simulink library "Library_SII"  (R2014b)
settings: Solver=ode45  StartTime=0.0  StopTime=10.0  RelTol=1e-3
libraries: fl_lib x77, Library_SII x44, nesl_utility x33, powerlib x15, mblibv1 x11, simulink x6, elec_lib x5, powerlib_extras x1
(part 3 of 4)

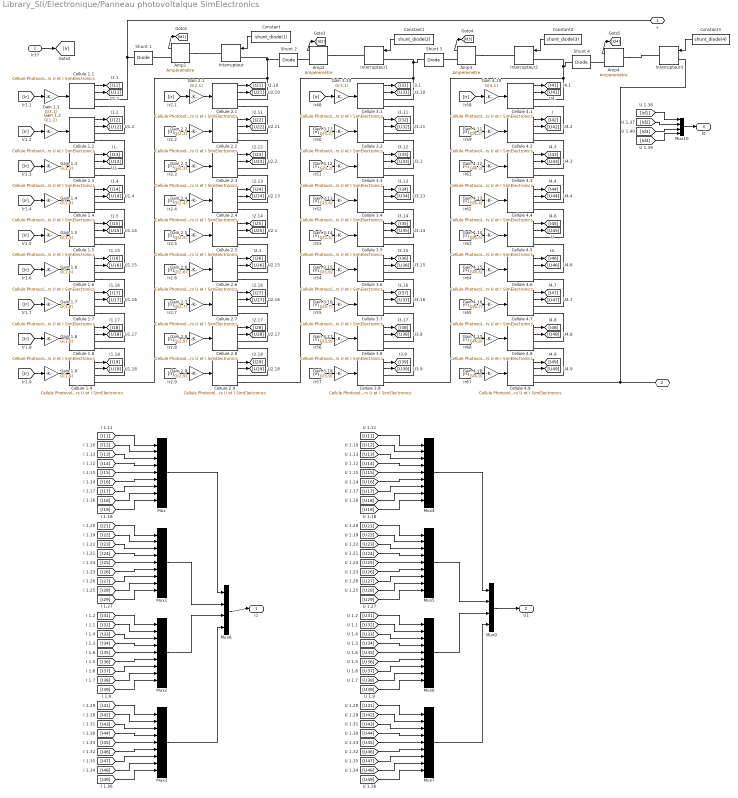
== system Library_SII/Electronique/Panneau photovoltaique SimElectronics ==
  Ir37 : Inport
  Amp{1..4} (4 alike) : Library_SII/Electronique/Ampèremètre
  Cellule 1.1 : Library_SII/Electronique/Cellule Photovoltaique avec capteurs U et I SimElectronics  typcell=polycristallin  Icc=Icc  Vco=Vco  Tcell=Tcell  shunt=0  mesure=off  IRef=1000  TRef=25  Qf=1.4
  Cellule 1.{2..8} (7 alike) : Library_SII/Electronique/Cellule Photovoltaique avec capteurs U et I SimElectronics  typcell=polycristallin  Icc=Icc  Vco=Vco  Tcell=Tcell  shunt=0  mesure=off  IRef=1000  TRef=25  Qf=1.5
  Cellule 1.9 : Library_SII/Electronique/Cellule Photovoltaique avec capteurs U et I SimElectronics  typcell=polycristallin  Icc=Icc  Vco=Vco  Tcell=Tcell  shunt=1  mesure=off  IRef=1000  TRef=25  Qf=1.5
  Cellule 2.{1..7} (7 alike) : Library_SII/Electronique/Cellule Photovoltaique avec capteurs U et I SimElectronics  typcell=polycristallin  Icc=Icc  Vco=Vco  Tcell=Tcell  shunt=0  mesure=off  IRef=1000  TRef=25  Qf=1.5
  Cellule 2.8 : Library_SII/Electronique/Cellule Photovoltaique avec capteurs U et I SimElectronics  typcell=polycristallin  Icc=Icc  Vco=Vco  Tcell=Tcell  shunt=0  mesure=off  IRef=1000  TRef=25  Qf=10
  Cellule 2.9 : Library_SII/Electronique/Cellule Photovoltaique avec capteurs U et I SimElectronics  typcell=polycristallin  Icc=Icc  Vco=Vco  Tcell=Tcell  shunt=1  mesure=off  IRef=1000  TRef=25  Qf=1.5
  Cellule 3.{1..8} (8 alike) : Library_SII/Electronique/Cellule Photovoltaique avec capteurs U et I SimElectronics  typcell=polycristallin  Icc=Icc  Vco=Vco  Tcell=Tcell  shunt=0  mesure=off  IRef=1000  TRef=25  Qf=1.5
  Cellule 3.9 : Library_SII/Electronique/Cellule Photovoltaique avec capteurs U et I SimElectronics  typcell=polycristallin  Icc=Icc  Vco=Vco  Tcell=Tcell  shunt=1  mesure=off  IRef=1000  TRef=25  Qf=1.5
  Cellule 4.{1..8} (8 alike) : Library_SII/Electronique/Cellule Photovoltaique avec capteurs U et I SimElectronics  typcell=polycristallin  Icc=Icc  Vco=Vco  Tcell=Tcell  shunt=0  mesure=off  IRef=1000  TRef=25  Qf=1.5
  Cellule 4.9 : Library_SII/Electronique/Cellule Photovoltaique avec capteurs U et I SimElectronics  typcell=polycristallin  Icc=Icc  Vco=Vco  Tcell=Tcell  shunt=1  mesure=off  IRef=1000  TRef=25  Qf=1.5
  Constant : Constant  Value=shunt_diode(1)
  Constant1 : Constant  Value=shunt_diode(2)
  Constant2 : Constant  Value=shunt_diode(3)
  Constant3 : Constant  Value=shunt_diode(4)
  Gain 1.1 : Gain  Gain=G(1,1)
  Gain 1.2 : Gain  Gain=G(1,2)
  Gain 1.3 : Gain  Gain=G(1,3)
  Gain 1.4 : Gain  Gain=G(1,4)
  Gain 1.5 : Gain  Gain=G(1,5)
  Gain 1.6 : Gain  Gain=G(1,6)
  Gain 1.7 : Gain  Gain=G(1,7)
  Gain 1.8 : Gain  Gain=G(1,8)
  Gain 1.9 : Gain  Gain=G(1,9)
  Gain 2.1 : Gain  Gain=G(2,1)
  Gain 2.2 : Gain  Gain=G(2,2)
  Gain 2.3 : Gain  Gain=G(2,3)
  Gain 2.4 : Gain  Gain=G(2,4)
  Gain 2.5 : Gain  Gain=G(2,5)
  Gain 2.6 : Gain  Gain=G(2,6)
  Gain 2.7 : Gain  Gain=G(2,7)
  Gain 2.8 : Gain  Gain=G(2,8)
  Gain 2.9 : Gain  Gain=G(2,9)
  Gain 3.10 : Gain  Gain=G(3,1)
  Gain 3.11 : Gain  Gain=G(3,2)
  Gain 3.12 : Gain  Gain=G(3,3)
  Gain 3.13 : Gain  Gain=G(3,4)
  Gain 3.14 : Gain  Gain=G(3,5)
  Gain 3.15 : Gain  Gain=G(3,6)
  Gain 3.16 : Gain  Gain=G(3,7)
  Gain 3.17 : Gain  Gain=G(3,8)
  Gain 3.18 : Gain  Gain=G(3,9)
  Gain 4.10 : Gain  Gain=G(4,1)
  Gain 4.11 : Gain  Gain=G(4,2)
  Gain 4.12 : Gain  Gain=G(4,3)
  Gain 4.13 : Gain  Gain=G(4,4)
  Gain 4.14 : Gain  Gain=G(4,5)
  Gain 4.15 : Gain  Gain=G(4,6)
  Gain 4.16 : Gain  Gain=G(4,7)
  Gain 4.17 : Gain  Gain=G(4,8)
  Gain 4.18 : Gain  Gain=G(4,9)
  Interrupteur{,1..3} (4 alike) : Library_SII/Electronique/Interrupteur
  Mux{,1..7} (8 alike) : Mux  Inputs=9
  Mux10 : Mux
  Mux8 : Mux
  Mux9 : Mux
  Shunt {1..4} (4 alike) : elec_lib/Semiconductor Devices/Diode  ModelType=1  Vf=0.6 V  Ron=0.3 Ohm  Goff=1e-8 S  Rz=0.3 Ohm  Vz=50 V  C_PWL=5 pF  prmExp=1  I12=[ 0.0137 0.545 ] A  V12=[ 0.6 0.7 ] V  I1=0.0137 A  V1=0.6 V  RS=0.01 Ohm  IS=1e-12 A  Tmeas=25 C  ec=1  BV=Inf V  C_param=1  CJ0=5 pF  VJ=1 V  Mgrad=0.5  Vvec=[ 0.1 10 100 ] V  Cvec=[ 3.5 1 0.4 ] pF  FC=0.5  Q_param=1  Irrm=-7.15 A  iF=4 A  didt=-750 A/us  trr=115 ns  TT=50 ns  tau=100 ns  T_param=1  IS_T2=1.25e-7 A  I1_T2=0.245 A  V1_T2=0.5 V  Tmeas2=125 C  EG_param=1  EG=1.11 eV  XTI_param=1  XTI=3  dBVdT=0 V/K  Tdevice=25 C  Rth=[ 0 10 ] K/W  thermal_mass_parameterization=1  thermal_mass=[ 0 1 ] J/K  thermal_time_constant=[ 0 10 ] s  thermal_mass_initial_temperatures=[ 25 25 ] C
  + : PMIOPort  Port=1  Side=Right
  - : PMIOPort  Port=2  Side=Right
  I1 : Outport
  U1 : Outport  Port=2
  Id : Outport  Port=3
  wires:
  Ir37/1 -> [Ir]
  [Ir] -> Gain 1.1/1
  Gain 1.1/1 -> Cellule 1.1/1
  Cellule 1.1/1 -> [I11]
  Cellule 1.1/2 -> [U11]
  [Ir] -> Gain 1.2/1
  Gain 1.2/1 -> Cellule 1.2/1
  Cellule 1.2/1 -> [I12]
  Cellule 1.2/2 -> [U12]
  [Ir] -> Gain 1.3/1
  Gain 1.3/1 -> Cellule 1.3/1
  Cellule 1.3/1 -> [I13]
  Cellule 1.3/2 -> [U13]
  [Ir] -> Gain 1.4/1
  Gain 1.4/1 -> Cellule 1.4/1
  Cellule 1.4/1 -> [I14]
  Cellule 1.4/2 -> [U14]
  [Ir] -> Gain 1.5/1
  Gain 1.5/1 -> Cellule 1.5/1
  Cellule 1.5/1 -> [I15]
  Cellule 1.5/2 -> [U15]
  [Ir] -> Gain 1.6/1
  Gain 1.6/1 -> Cellule 1.6/1
  Cellule 1.6/1 -> [I16]
  Cellule 1.6/2 -> [U16]
  [Ir] -> Gain 1.7/1
  Gain 1.7/1 -> Cellule 1.7/1
  Cellule 1.7/1 -> [I17]
  Cellule 1.7/2 -> [U17]
  [Ir] -> Gain 1.8/1
  Gain 1.8/1 -> Cellule 1.8/1
  Cellule 1.8/1 -> [I18]
  Cellule 1.8/2 -> [U18]
  [Ir] -> Gain 1.9/1
  Gain 1.9/1 -> Cellule 1.9/1
  Cellule 1.9/1 -> [I19]
  Cellule 1.9/2 -> [U19]
  [Ir] -> Gain 2.1/1
  Gain 2.1/1 -> Cellule 2.1/1
  Cellule 2.1/1 -> [I21]
  Cellule 2.1/2 -> [U21]
  [Ir] -> Gain 2.2/1
  Gain 2.2/1 -> Cellule 2.2/1
  Cellule 2.2/1 -> [I22]
  Cellule 2.2/2 -> [U22]
  [Ir] -> Gain 2.3/1
  Gain 2.3/1 -> Cellule 2.3/1
  Cellule 2.3/1 -> [I23]
  Cellule 2.3/2 -> [U23]
  [Ir] -> Gain 2.4/1
  Gain 2.4/1 -> Cellule 2.4/1
  Cellule 2.4/1 -> [I24]
  Cellule 2.4/2 -> [U24]
  [Ir] -> Gain 2.5/1
  Gain 2.5/1 -> Cellule 2.5/1
  Cellule 2.5/1 -> [I25]
  Cellule 2.5/2 -> [U25]
  [Ir] -> Gain 2.6/1
  Gain 2.6/1 -> Cellule 2.6/1
  Cellule 2.6/1 -> [I26]
  Cellule 2.6/2 -> [U26]
  [Ir] -> Gain 2.7/1
  Gain 2.7/1 -> Cellule 2.7/1
  Cellule 2.7/1 -> [I27]
  Cellule 2.7/2 -> [U27]
  [Ir] -> Gain 2.8/1
  Gain 2.8/1 -> Cellule 2.8/1
  Cellule 2.8/1 -> [I28]
  Cellule 2.8/2 -> [U28]
  [Ir] -> Gain 2.9/1
  Gain 2.9/1 -> Cellule 2.9/1
  Cellule 2.9/1 -> [I29]
  Cellule 2.9/2 -> [U29]
  [Ir] -> Gain 3.10/1
  Gain 3.10/1 -> Cellule 3.1/1
  Cellule 3.1/1 -> [I31]
  Cellule 3.1/2 -> [U31]
  [Ir] -> Gain 3.11/1
  Gain 3.11/1 -> Cellule 3.2/1
  Cellule 3.2/1 -> [I32]
  Cellule 3.2/2 -> [U32]
  [Ir] -> Gain 3.12/1
  Gain 3.12/1 -> Cellule 3.3/1
  Cellule 3.3/1 -> [I33]
  Cellule 3.3/2 -> [U33]
  [Ir] -> Gain 3.13/1
  Gain 3.13/1 -> Cellule 3.4/1
  Cellule 3.4/1 -> [I34]
  Cellule 3.4/2 -> [U34]
  [Ir] -> Gain 3.14/1
  Gain 3.14/1 -> Cellule 3.5/1
  Cellule 3.5/1 -> [I35]
  Cellule 3.5/2 -> [U35]
  [Ir] -> Gain 3.15/1
  Gain 3.15/1 -> Cellule 3.6/1
  Cellule 3.6/1 -> [I36]
  Cellule 3.6/2 -> [U36]
  [Ir] -> Gain 3.16/1
  Gain 3.16/1 -> Cellule 3.7/1
  Cellule 3.7/1 -> [I37]
  Cellule 3.7/2 -> [U37]
  [Ir] -> Gain 3.17/1
  Gain 3.17/1 -> Cellule 3.8/1
  Cellule 3.8/1 -> [I38]
  Cellule 3.8/2 -> [U38]
  [Ir] -> Gain 3.18/1
  Gain 3.18/1 -> Cellule 3.9/1
  Cellule 3.9/1 -> [I39]
  Cellule 3.9/2 -> [U39]
  [Ir] -> Gain 4.10/1
  Gain 4.10/1 -> Cellule 4.1/1
  Cellule 4.1/1 -> [I41]
  Cellule 4.1/2 -> [U41]
  [Ir] -> Gain 4.11/1
  Gain 4.11/1 -> Cellule 4.2/1
  Cellule 4.2/1 -> [I42]
  Cellule 4.2/2 -> [U42]
  [Ir] -> Gain 4.12/1
  Gain 4.12/1 -> Cellule 4.3/1
  Cellule 4.3/1 -> [I43]
  Cellule 4.3/2 -> [U43]
  [Ir] -> Gain 4.13/1
  Gain 4.13/1 -> Cellule 4.4/1
  Cellule 4.4/1 -> [I44]
  Cellule 4.4/2 -> [U44]
  [Ir] -> Gain 4.14/1
  Gain 4.14/1 -> Cellule 4.5/1
  Cellule 4.5/1 -> [I45]
  Cellule 4.5/2 -> [U45]
  [Ir] -> Gain 4.15/1
  Gain 4.15/1 -> Cellule 4.6/1
  Cellule 4.6/1 -> [I46]
  Cellule 4.6/2 -> [U46]
  [Ir] -> Gain 4.16/1
  Gain 4.16/1 -> Cellule 4.7/1
  Cellule 4.7/1 -> [I47]
  Cellule 4.7/2 -> [U47]
  [Ir] -> Gain 4.17/1
  Gain 4.17/1 -> Cellule 4.8/1
  Cellule 4.8/1 -> [I48]
  Cellule 4.8/2 -> [U48]
  [Ir] -> Gain 4.18/1
  Gain 4.18/1 -> Cellule 4.9/1
  Cellule 4.9/1 -> [I49]
  Cellule 4.9/2 -> [U49]
  [I11] -> Mux/1
  [I12] -> Mux/2
  [I13] -> Mux/3
  [I14] -> Mux/4
  [I15] -> Mux/5
  [I19] -> Mux/9
  [I18] -> Mux/8
  [I17] -> Mux/7
  [I16] -> Mux/6
  [I25] -> Mux1/5
  [I21] -> Mux1/1
  [I22] -> Mux1/2
  [I23] -> Mux1/3
  [I24] -> Mux1/4
  [I26] -> Mux1/6
  [I29] -> Mux1/9
  [I28] -> Mux1/8
  [I27] -> Mux1/7
  [I35] -> Mux2/5
  [I45] -> Mux3/5
  [U15] -> Mux4/5
  [U25] -> Mux5/5
  [U35] -> Mux6/5
  [U45] -> Mux7/5
  Mux1/1 -> Mux8/2
  Mux/1 -> Mux8/1
  Mux2/1 -> Mux8/3
  Mux3/1 -> Mux8/4
  Mux5/1 -> Mux9/2
  Mux4/1 -> Mux9/1
  Mux6/1 -> Mux9/3
  Mux7/1 -> Mux9/4
  [I31] -> Mux2/1
  [I39] -> Mux2/9
  [I38] -> Mux2/8
  [I37] -> Mux2/7
  [I36] -> Mux2/6
  [I32] -> Mux2/2
  [I33] -> Mux2/3
  [I34] -> Mux2/4
  [I41] -> Mux3/1
  [I42] -> Mux3/2
  [I43] -> Mux3/3
  [I49] -> Mux3/9
  [I48] -> Mux3/8
  [I47] -> Mux3/7
  [I46] -> Mux3/6
  [I44] -> Mux3/4
  [U11] -> Mux4/1
  [U19] -> Mux4/9
  [U21] -> Mux5/1
  [U29] -> Mux5/9
  [U31] -> Mux6/1
  [U39] -> Mux6/9
  [U41] -> Mux7/1
  [U49] -> Mux7/9
  [U12] -> Mux4/2
  [U13] -> Mux4/3
  [U14] -> Mux4/4
  [U16] -> Mux4/6
  [U18] -> Mux4/8
  [U17] -> Mux4/7
  [U22] -> Mux5/2
  [U23] -> Mux5/3
  [U24] -> Mux5/4
  [U28] -> Mux5/8
  [U27] -> Mux5/7
  [U26] -> Mux5/6
  [U32] -> Mux6/2
  [U33] -> Mux6/3
  [U34] -> Mux6/4
  [U38] -> Mux6/8
  [U37] -> Mux6/7
  [U36] -> Mux6/6
  [U42] -> Mux7/2
  [U43] -> Mux7/3
  [U44] -> Mux7/4
  [U48] -> Mux7/8
  [U47] -> Mux7/7
  [U46] -> Mux7/6
  Mux8/1 -> I1/1
  Mux9/1 -> U1/1
  Mux10/1 -> Id/1
  Constant/1 -> Interrupteur/1
  Amp1/1 -> [Id1]
  Constant1/1 -> Interrupteur1/1
  Amp2/1 -> [Id2]
  Constant2/1 -> Interrupteur2/1
  Amp3/1 -> [Id3]
  Constant3/1 -> Interrupteur3/1
  Amp4/1 -> [Id4]
  [Id1] -> Mux10/1
  [Id2] -> Mux10/2
  [Id3] -> Mux10/3
  [Id4] -> Mux10/4
  connections:
  Cellule 2.1/RConn2 -- Cellule 2.2/RConn1
  Cellule 3.8/RConn2 -- Cellule 3.9/RConn1
  Cellule 3.6/RConn2 -- Cellule 3.7/RConn1
  Cellule 4.3/RConn2 -- Cellule 4.4/RConn1
  Cellule 3.4/RConn2 -- Cellule 3.5/RConn1
  Cellule 4.1/RConn2 -- Cellule 4.2/RConn1
  Cellule 3.2/RConn2 -- Cellule 3.3/RConn1
  Cellule 4.2/RConn2 -- Cellule 4.3/RConn1
  Cellule 3.3/RConn2 -- Cellule 3.4/RConn1
  Cellule 3.7/RConn2 -- Cellule 3.8/RConn1
  Cellule 3.5/RConn2 -- Cellule 3.6/RConn1
  Cellule 3.1/RConn2 -- Cellule 3.2/RConn1
  +/RConn1 -- Cellule 1.1/RConn1 -- Shunt 1/RConn1
  Cellule 2.4/RConn2 -- Cellule 2.5/RConn1
  Cellule 2.5/RConn2 -- Cellule 2.6/RConn1
  Cellule 2.2/RConn2 -- Cellule 2.3/RConn1
  Cellule 2.3/RConn2 -- Cellule 2.4/RConn1
  Cellule 2.6/RConn2 -- Cellule 2.7/RConn1
  Cellule 1.1/RConn2 -- Cellule 1.2/RConn1
  Cellule 1.4/RConn2 -- Cellule 1.5/RConn1
  Cellule 1.2/RConn2 -- Cellule 1.3/RConn1
  Cellule 1.6/RConn2 -- Cellule 1.7/RConn1
  Cellule 1.7/RConn2 -- Cellule 1.8/RConn1
  Cellule 1.5/RConn2 -- Cellule 1.6/RConn1
  Cellule 1.8/RConn2 -- Cellule 1.9/RConn1
  Cellule 1.3/RConn2 -- Cellule 1.4/RConn1
  Cellule 2.7/RConn2 -- Cellule 2.8/RConn1
  Cellule 2.8/RConn2 -- Cellule 2.9/RConn1
  Cellule 4.4/RConn2 -- Cellule 4.5/RConn1
  Cellule 4.5/RConn2 -- Cellule 4.6/RConn1
  Cellule 4.6/RConn2 -- Cellule 4.7/RConn1
  Cellule 4.7/RConn2 -- Cellule 4.8/RConn1
  Cellule 4.8/RConn2 -- Cellule 4.9/RConn1
  -/RConn1 -- Cellule 4.9/RConn2 -- Interrupteur3/LConn1
  Cellule 2.1/RConn1 -- Shunt 2/RConn1 -- Interrupteur/LConn1 -- Cellule 1.9/RConn2
  Cellule 2.9/RConn2 -- Shunt 3/RConn1 -- Interrupteur1/LConn1 -- Cellule 3.1/RConn1
  Cellule 3.9/RConn2 -- Shunt 4/RConn1 -- Interrupteur2/LConn1 -- Cellule 4.1/RConn1
  Amp1/RConn1 -- Shunt 1/LConn1
  Amp1/LConn1 -- Interrupteur/RConn1
  Amp2/RConn1 -- Shunt 2/LConn1
  Amp2/LConn1 -- Interrupteur1/RConn1
  Amp3/RConn1 -- Shunt 3/LConn1
  Amp3/LConn1 -- Interrupteur2/RConn1
  Amp4/RConn1 -- Shunt 4/LConn1
  Amp4/LConn1 -- Interrupteur3/RConn1

== system Library_SII/Electronique/Simscape<->SPS ==
  Controlled Current Source : powerlib/Electrical Sources/Controlled Current Source  Initialize=on  Source_Type=AC  Amplitude=0  Phase=0  Frequency=0  Measurements=None
  Controlled Voltage Source : fl_lib/Electrical/Electrical Sources/Controlled Voltage Source
  Current Sensor : fl_lib/Electrical/Electrical Sensors/Current Sensor
  PS-S I : nesl_utility/PS-Simulink Converter  PhysicalDomain=network_engine_domain  SubClassName=ps_output  LeftPortType=input  RightPortType=output  PseudoPeriodic=off  Frequencies=[]  Unit=1  AffineConversion=off
  S-PS V : nesl_utility/Simulink-PS Converter  PhysicalDomain=network_engine_domain  SubClassName=ps_input  LeftPortType=input  RightPortType=output  PseudoPeriodic=off  Frequencies=[]  NoiseDistribution=none  NoiseParameters=[]  Unit=1  AffineConversion=off  InputFiltering=off  SimscapeFilterOrder=1  InputFilterTimeConstant=.001  UdotUserProvided=0
  Series RLC Branch : powerlib/Elements/Series RLC Branch  LConnTagsString=__new0  RConnTagsString=__new0  BranchType=R  Resistance=1e12  Inductance=1e-3  SetiL0=off  InitialCurrent=0  Capacitance=1e-6  Setx0=off  InitialVoltage=0  Measurements=None
  Voltage Measurement : powerlib/Measurements/Voltage Measurement  PhasorSimulation=off  OutputType=Complex  PSBequivalent=0
  SPS + : PMIOPort  Port=1  Side=Right
  SS + : PMIOPort  Port=2  Side=Left
  SPS - : PMIOPort  Port=3  Side=Right
  SS - : PMIOPort  Port=4  Side=Left
  wires:
  PS-S I/1 -> Controlled Current Source/1
  Voltage Measurement/1 -> S-PS V/1
  connections:
  SS -/RConn1 -- Controlled Voltage Source/RConn2
  SPS -/RConn1 -- Voltage Measurement/LConn2
  SS +/RConn1 -- Current Sensor/LConn1
  Series RLC Branch/RConn1 -- Controlled Current Source/RConn1 -- SPS +/RConn1
  PS-S I/LConn1 -- Current Sensor/RConn1
  S-PS V/RConn1 -- Controlled Voltage Source/RConn1
  Current Sensor/RConn2 -- Controlled Voltage Source/LConn1
  Series RLC Branch/LConn1 -- Controlled Current Source/LConn1 -- Voltage Measurement/LConn1

== system Library_SII/Electronique/Voltmètre ==
  PS-Simulink Converter1 : nesl_utility/PS-Simulink Converter  PhysicalDomain=network_engine_domain  SubClassName=ps_output  LeftPortType=input  RightPortType=output  PseudoPeriodic=off  Frequencies=[]  Unit=1  AffineConversion=off
  Voltage Sensor : fl_lib/Electrical/Electrical Sensors/Voltage Sensor
  Conn1 : PMIOPort  Port=1  Side=Left
  Conn2 : PMIOPort  Port=2  Side=Right
  Out1 : Outport
  wires:
  PS-Simulink Converter1/1 -> Out1/1
  connections:
  Voltage Sensor/RConn1 -- PS-Simulink Converter1/LConn1
  Conn1/RConn1 -- Voltage Sensor/LConn1
  Conn2/RConn1 -- Voltage Sensor/RConn2

== system Library_SII/Mécanique/Capteur de puissance mécanique de rotation ==
  Ideal Rotational Motion Sensor : fl_lib/Mechanical/Mechanical Sensors/Ideal Rotational Motion Sensor  offset=0 rad
  Ideal Torque Sensor : fl_lib/Mechanical/Mechanical Sensors/Ideal Torque Sensor
  PS-Simulink Converter : nesl_utility/PS-Simulink Converter  PhysicalDomain=network_engine_domain  SubClassName=ps_output  LeftPortType=input  RightPortType=output  PseudoPeriodic=off  Frequencies=[]  Unit=1  AffineConversion=off
  PS-Simulink Converter1 : nesl_utility/PS-Simulink Converter  PhysicalDomain=network_engine_domain  SubClassName=ps_output  LeftPortType=input  RightPortType=output  PseudoPeriodic=off  Frequencies=[]  Unit=1  AffineConversion=off
  Product : Product  RndMeth=Zero
  Ref : PMIOPort  Tag=PMCPort  Port=1  Side=Left
  E : PMIOPort  Port=2  Side=Left
  S : PMIOPort  Tag=PMCPort  Port=3  Side=Right
  P : Outport
  C : Outport  Port=2
  W : Outport  Port=3
  wires:
  PS-Simulink Converter/1 -> C/1, Product/1
  PS-Simulink Converter1/1 -> W/1, Product/2
  Product/1 -> P/1
  connections:
  Ideal Torque Sensor/LConn1 -- E/RConn1
  Ideal Torque Sensor/RConn1 -- S/RConn1 -- Ideal Rotational Motion Sensor/RConn1
  Ideal Rotational Motion Sensor/LConn1 -- Ref/RConn1
  Ideal Rotational Motion Sensor/RConn2 -- PS-Simulink Converter1/LConn1
  Ideal Torque Sensor/RConn2 -- PS-Simulink Converter/LConn1

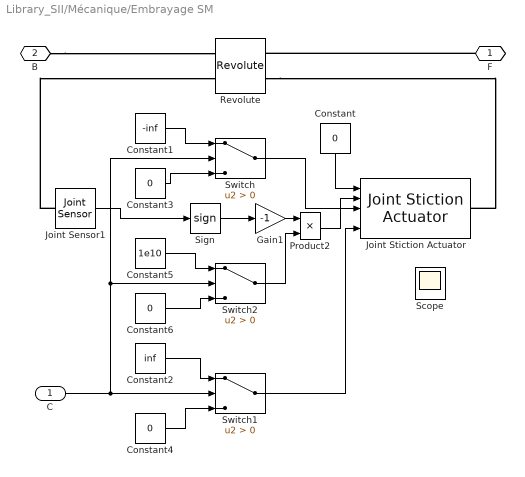
== system Library_SII/Mécanique/Embrayage SM ==
  C : Inport
  Constant{,3..4,6} (4 alike) : Constant  Value=0
  Constant1 : Constant  Value=-inf
  Constant2 : Constant  Value=inf
  Constant5 : Constant  Value=1e10
  Gain1 : Gain  Gain=-1  SaturateOnIntegerOverflow=on  OutDataTypeStr=Inherit: Same as input  ParamDataTypeStr=Inherit: Same as input
  Joint Sensor1 : mblibv1/Sensors &  Actuators/Joint Sensor  UpdateFromCAD=off  PhysicalDomain=Mechanical  PortType=blob  Muxed=off  Pose=off  Angle=off  AngleUnits=deg  ArcVelocity=on  ArcVelocityUnits=rad/s  ArcAcceleration=off  ArcAccelerationUnits=deg/s^2  CoordPosition=on  CoordPositionUnits=m  Velocity=off  VelocityUnits=m/s  Acceleration=off  AccelerationUnits=m/s^2  Quaternion=on  QuaternionDT=off  QuaternionDDT=off  QuaternionUnits=off  OutputVector=[1]  ActiveIO=on  Width=1  DialogClass=MechanicalSensorBlock  Primitive=R1  Force=off  ForceUnits=N  Torque=off  TorqueUnits=N*m  ReferenceFrame=Absolute (World)  ReactionSensedSide=Base  ReactionReferenceFrame=Absolute (World)  ReactionForce=off  ReactionForceUnits=N  ReactionMoment=off  ReactionMomentUnits=N*m
  Joint Stiction Actuator : mblibv1/Sensors &  Actuators/Joint Stiction Actuator  UpdateFromCAD=off  PhysicalDomain=Mechanical  PortType=blob  ActuationStyle=Force  AngleUnits=deg  ArcVelocityUnits=deg/s  ArcAccelerationUnits=deg/s^2  CoordPositionUnits=m  VelocityUnits=m/s  AccelerationUnits=m/s^2  ForceUnits=N  TorqueUnits=N-m  ActiveIO=on  Width=5  DialogClass=EventActuatorBlock  Primitive=R1  FrictionalForceUnits=N  ExternalForceUnits=N  FrictionalTorqueUnits=N*m  ExternalTorqueUnits=N*m  LockingTolerance=1e-2
  Product2 : Product  SaturateOnIntegerOverflow=on  InputSameDT=on  OutDataTypeStr=Inherit: Same as first input
  Revolute : mblibv1/Joints/Revolute  LConnTagsString=__newl0|SA1  RConnTagsString=__newr0|SA1  UpdateFromCAD=off  NumSAPorts=2  CutJoint=off  MarkAsCut=off  Primitives=prismatic  PrimitiveProps=R1$World$axe$revolute  DialogClass=JointBlock  R1Axis=axe
  Scope : Scope
  Sign : Signum  ZeroCross=off
  Switch : Switch  Criteria=u2 > Threshold
  Switch1 : Switch  Criteria=u2 > Threshold
  Switch2 : Switch  Criteria=u2 > Threshold
  F : PMIOPort  Port=1  Side=Right
  B : PMIOPort  Port=2  Side=Left
  wires:
  Switch2/1 -> Product2/2
  Product2/1 -> Joint Stiction Actuator/2
  Gain1/1 -> Product2/1
  Sign/1 -> Gain1/1
  Joint Sensor1/1 -> Sign/1
  Constant5/1 -> Switch2/1
  Constant6/1 -> Switch2/3
  Constant2/1 -> Switch1/1
  Constant4/1 -> Switch1/3
  Constant1/1 -> Switch/1
  Constant3/1 -> Switch/3
  C/1 -> Switch2/2, Switch/2, Switch1/2
  Switch1/1 -> Joint Stiction Actuator/5
  Switch/1 -> Joint Stiction Actuator/3
  Constant/1 -> Joint Stiction Actuator/1
  connections:
  B/RConn1 -- Revolute/LConn1
  F/RConn1 -- Revolute/RConn1
  Revolute/RConn2 -- Joint Stiction Actuator/RConn1
  Joint Sensor1/LConn1 -- Revolute/LConn2

== system Library_SII/Mécanique/Engrenage droit SS ==
  Capteur de puissance mécanique de rotation : Subsystem  mask(Capteur de puissance mécanique de rotation){}
      mask help:
      | Le bloc représente un capteur de puissance mécanique de rotation.
      | R et C sont des ports physiques conservatifs.
      |
      | P, T et W sont des ports Simulink délivrant les valeurs de :
      |  - la puissance mécanique traversant le bloc (en W)
      |  - le couple transmis à travers le bloc (en Nm)
      |  - la vitesse de rotation (en rad/s)
      |
      | Ces valeurs sont calculées par rapport au référentiel Ref.
      mask Display:
      | plot([149.600878633536;150.016472378793;150.47508104106;150.972287968219;151.50330478576;152.063017511447;152.646035805762;153.246744883819;153.859359588817;154.477980106257;155.096648782383;155.709407499646;156.310355056631;156.893703999851;157.453836360095;157.985357756531;158.483149347555;158.942417128023;159.358738098149;159.728102859405;160.046954227227;160.312221488639;160.521349974904;160.672325664379;160.763694578642;160.794576785101;160.764674871227;160.674276808796;160.524253180566;160.316048796087;160.051668777399;159.733659248606;159.365082815313;158.949489070056;158.490880407788;157.993673480629;157.462656663088;156.908284800231], [156.971389291536;157.430657072004;157.84697804213;158.216342803387;158.535194171208;158.80046143262;159.009589918885;159.16056560836;159.251934522623;159.282816729083;159.252914815208;159.162516752777;159.012493124547;158.804288740068;158.53990872138;158.221899192587;157.853322759294;157.437729014037;156.979120351769;156.48191342461;155.950896607069;155.391183881382;154.808165587067;154.20745650901;153.594841804012;152.976221286573;152.357552610446;151.744793893183;151.143846336199;150.560497392978;150.000365032735;149.468843636298;148.971052045274;148.511784264806;148.095463294681;147.726098533424;147.407247165603;147.144199990631])
      | plot([152.057635404444;152.93604260309;153.834625296826;154.744729643097;155.657590839533;156.564417533794;157.45647648909;158.325176690034;159.162152078811;159.959342124889;160.709069452336;161.404113777147;162.037781442523;162.603969882449;163.097226392739;163.512800643557;163.846690427691;164.095680203997;164.257372064819;164.330208829146;164.313489039122;164.27939575172], [142.228020686971;141.979030910664;141.817339049842;141.744502285515;141.761222075539;141.867337399197;142.061826307913;142.342815767178;142.707599694895;143.152665022428;143.673725527376;144.265763112236;144.923076131425;145.639334301243;146.40763966397;147.220593018964;148.070365181011;148.948772379657;149.847355073393;150.757459419663;151.6703206161;152.055850472277])
      | %plot([116.468514315784;116.438789536125;116.349901463023;116.202706137216;115.998621130155;115.739611892022;115.42817282337;115.067303252679;114.660478551187;114.211616663162;113.725040373958;113.205435679231;112.657806656235;112.087427271827;111.499790591278;110.900555877058;110.29549408704;109.690432297022;109.091197582803;108.503560902254;107.933181517846;107.38555249485;106.865947800123;106.379371510919;105.930509622894;105.523684921402;105.162815350711;104.851376282059;104.592367043926;104.388282036865;104.241086711057;104.152198637956;104.122473858297;104.152198637956;104.241086711057;104.388282036865;104.592367043926;104.851376282059;105.162815350711;105.523684921402;105.930509622894;106.379371510919;106.865947800123;107.38555249485;107.933181517846;108.503560902254;109.091197582803;109.690432297022;110.29549408704;110.900555877058;111.499790591278;112.087427271827;112.657806656235;113.205435679231;113.725040373958;114.211616663162;114.660478551187;115.067303252679;115.42817282337;115.739611892022;115.998621130155;116.202706137216;116.349901463023;116.438789536125;116.468514315784;116.468514315784], [111.618284136057;111.013222346039;110.413987631819;109.826350951271;109.255971566862;108.708342543866;108.188737849139;107.702161559936;107.253299671911;106.846474970419;106.485605399728;106.174166331075;105.915157092943;105.711072085881;105.563876760074;105.474988686973;105.445263907313;105.474988686973;105.563876760074;105.711072085881;105.915157092943;106.174166331075;106.485605399728;106.846474970419;107.253299671911;107.702161559936;108.188737849139;108.708342543866;109.255971566862;109.826350951271;110.413987631819;111.013222346039;111.618284136057;112.223345926075;112.822580640295;113.410217320843;113.980596705252;114.528225728247;115.047830422975;115.534406712178;115.983268600203;116.390093301695;116.750962872386;117.062401941038;117.321411179171;117.525496186232;117.67269151204;117.761579585141;117.7913043648;117.761579585141;117.67269151204;117.525496186232;117.321411179171;117.062401941038;116.750962872386;116.390093301695;115.983268600203;115.534406712178;115.047830422975;114.528225728247;113.980596705252;113.410217320843;112.822580640295;112.223345926075;111.618284136057;111.618284136057])
      | plot([239.23602886498;238.828071429858;237.608127977604;235.587947230552;232.78698463364;229.232214987837;224.957872668068;220.005121927465;214.421660463109;208.261260061133;201.583248745024;194.451939414329;186.936010476274;179.107844435155;171.042830809261;162.818640088593;154.514475725591;146.210311362589;137.986120641921;129.921107016027;122.092940974909;114.577012036853;107.445702706158;100.76769139005;94.607290988073;89.0238295237172;84.0710787831142;79.7967364633452;76.2419668175427;73.4410042206305;71.4208234735788;70.2008800213248;69.7929225862026;70.2008800213248;71.4208234735788;73.4410042206306;76.2419668175428;79.7967364633454;84.0710787831144;89.0238295237174;94.6072909880733;100.76769139005;107.445702706159;114.577012036853;122.092940974909;129.921107016027;137.986120641921;146.210311362589;154.514475725591;162.818640088593;171.042830809261;179.107844435155;186.936010476274;194.451939414329;201.583248745024;208.261260061133;214.421660463109;220.005121927465;224.957872668068;229.232214987837;232.78698463364;235.587947230552;237.608127977604;238.828071429858;239.23602886498;239.23602886498], [155.774275772274;147.47628550917;139.258209428443;131.199192095207;123.376846251889;115.866505365088;108.740498123116;102.067451871182;95.9116316925529;90.3323215006612;85.3832531026163;81.1120887325275;77.5599620381344;74.7610819412943;72.742403187363;71.5233667562631;71.1157126352191;71.5233667562631;72.742403187363;74.7610819412943;77.5599620381345;81.1120887325275;85.3832531026164;90.3323215006612;95.9116316925529;102.067451871182;108.740498123116;115.866505365089;123.376846251889;131.199192095207;139.258209428443;147.47628550917;155.774275772274;164.072266035377;172.290342116104;180.34935944934;188.171705292658;195.682046179459;202.808053421432;209.481099673365;215.636919851994;221.216230043886;226.165298441931;230.43646281202;233.988589506413;236.787469603253;238.806148357184;240.025184788284;240.432838909328;240.025184788284;238.806148357184;236.787469603253;233.988589506413;230.43646281202;226.165298441931;221.216230043886;215.636919851994;209.481099673365;202.808053421432;195.682046179459;188.171705292658;180.34935944934;172.290342116105;164.072266035378;155.774275772274;155.774275772274])
      | plot([252.715889364481;252.243022716633;250.828976737403;248.487369462568;245.240751850236;241.120390602797;236.165967051481;230.425195003451;223.953361231755;216.812793033479;209.072257983804;200.806301666664;192.094529760025;183.020841389688;173.672621134841;164.139897466795;154.514475725591;144.889053984387;135.356330316341;126.008110061494;116.934421691157;108.222649784518;99.9566934673787;92.2161584177032;85.075590219427;78.6037564477313;72.8629843997015;67.9085608483856;63.7881996009461;60.5415819886144;58.199974713779;56.7859287345493;56.3130620867014;56.7859287345493;58.1999747137791;60.5415819886146;63.7881996009463;67.9085608483858;72.8629843997018;78.6037564477315;85.0755902194273;92.2161584177035;99.9566934673791;108.222649784519;116.934421691157;126.008110061494;135.356330316341;144.889053984387;154.514475725591;164.139897466796;173.672621134841;183.020841389688;192.094529760025;200.806301666664;209.072257983803;216.812793033479;223.953361231755;230.425195003451;236.165967051481;241.120390602797;245.240751850236;248.487369462568;250.828976737403;252.243022716633;252.715889364481;252.715889364481], [154.514475725591;144.895228084285;135.36861905618;126.026395093992;116.958526921455;108.252343066071;99.9916888376535;92.2561188521535;85.1201308772245;78.6524483779929;72.9153586725213;67.9641130708855;63.8463947748555;60.6018596625959;58.2617543808809;56.8486154228053;56.3760520890355;56.8486154228053;58.2617543808809;60.6018596625959;63.8463947748555;67.9641130708856;72.9153586725213;78.652448377993;85.1201308772246;92.2561188521536;99.9916888376536;108.252343066072;116.958526921455;126.026395093992;135.36861905618;144.895228084285;154.514475725591;164.133723366898;173.660332395002;183.002556357191;192.070424529728;200.776608385111;209.037262613529;216.772832599029;223.908820573958;230.37650307319;236.113592778661;241.064838380297;245.182556676327;248.427091788587;250.767197070302;252.180336028377;252.652899362147;252.180336028377;250.767197070301;248.427091788587;245.182556676327;241.064838380297;236.113592778661;230.37650307319;223.908820573958;216.772832599029;209.037262613529;200.776608385111;192.070424529728;183.002556357191;173.660332395002;164.133723366898;154.514475725592;154.514475725591])
      | plot([154.514475725591;129.948374815285;179.017586633563;154.514475725591], [240.369848906994;203.583687543869;203.583687543869;240.369848906994])
      | %plot([105.382273904979;149.60125554353], [115.271704271436;156.971085816622])
      | plot([144.688035361469;144.688035361469], [152.057865634561;203.583687543869])
      | plot([164.277926087379;164.277926087379], [152.057865634561;203.583687543869])
      | plot([159.112745895982;159.616665914655], [149.60125554353;149.60125554353])
      | %plot([115.208714269102;159.364705905318], [107.901873998344;149.60125554353])
      | plot([0;311.800511553884;311.800511553884;0;0], [311.800511553884;311.800511553884;0;0;311.800511553884])
      | ;
      | color('red');
      | port_label('LConn', 1,'R')
      | port_label('RConn', 1,'C')
      | port_label('LConn', 2,'Ref')
      | port_label('output', 1,'P')
      | port_label('output', 2,'T')
      | port_label('output', 3,'W')
      | %port_label('RConn', 3,'A')
  Couple d'entrée : Scope
      settings: TimeRange=4  YMin=-0.5005000000000001  YMax=-0.4985000000000001  SaveName=ScopeData2
  Couple de sortie : Scope
      settings: TimeRange=4  YMin=-0.1  YMax=0
  Gain : Gain  Gain=1-n
  Gear Box : fl_lib/Mechanical/Mechanisms/Gear Box  ratio=r  t_in_specify=off  t_in_priority=High  t_in=0 N*m  t_out_specify=off  t_out_priority=High  t_out=0 N*m
  Ideal Torque Source : fl_lib/Mechanical/Mechanical Sources/Ideal Torque Source
  Inertia : fl_lib/Mechanical/Rotational Elements/Inertia  inertia=J kg*m^2  w_specify=on  w_priority=High  w=0 rad/s  t_specify=off  t_priority=High  t=0 N*m
  Simulink-PS Converter : nesl_utility/Simulink-PS Converter  PhysicalDomain=network_engine_domain  SubClassName=ps_input  LeftPortType=input  RightPortType=output  PseudoPeriodic=off  Frequencies=[]  NoiseDistribution=none  NoiseParameters=[]  Unit=1  AffineConversion=off  InputFiltering=off  SimscapeFilterOrder=1  InputFilterTimeConstant=.001  UdotUserProvided=0
  R : PMIOPort  Port=1  Side=Right
  V : PMIOPort  Tag=PMCPort  Port=2  Side=Left
  Ref : PMIOPort  Tag=PMCPort  Port=3  Side=Left
  wires:
  Capteur de puissance mécanique de rotation/2(C) -> Gain/1, Couple d'entrée/1
  Gain/1 -> Simulink-PS Converter/1, Couple de sortie/1
  connections:
  V/RConn1 -- Capteur de puissance mécanique de rotation/LConn2
  Capteur de puissance mécanique de rotation/LConn1 -- Ideal Torque Source/RConn2 -- Ref/RConn1
  R/RConn1 -- Gear Box/RConn1
  Simulink-PS Converter/RConn1 -- Ideal Torque Source/RConn1
  Inertia/LConn1 -- Gear Box/LConn1 -- Ideal Torque Source/LConn1 -- Capteur de puissance mécanique de rotation/RConn1

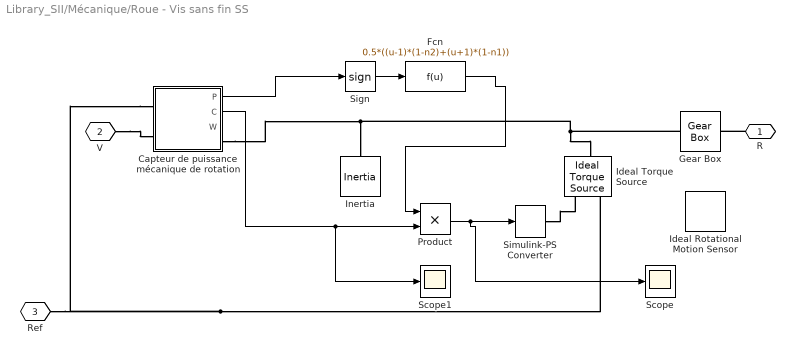
== system Library_SII/Mécanique/Roue - Vis sans fin SS ==
  Capteur de puissance mécanique de rotation : Subsystem  mask(Capteur de puissance mécanique de rotation){}
      mask help:
      | Le bloc représente un capteur de puissance mécanique de rotation.
      | R et C sont des ports physiques conservatifs.
      |
      | P, T et W sont des ports Simulink délivrant les valeurs de :
      |  - la puissance mécanique traversant le bloc (en W)
      |  - le couple transmis à travers le bloc (en Nm)
      |  - la vitesse de rotation (en rad/s)
      |
      | Ces valeurs sont calculées par rapport au référentiel Ref.
      mask Display:
      | plot([149.600878633536;150.016472378793;150.47508104106;150.972287968219;151.50330478576;152.063017511447;152.646035805762;153.246744883819;153.859359588817;154.477980106257;155.096648782383;155.709407499646;156.310355056631;156.893703999851;157.453836360095;157.985357756531;158.483149347555;158.942417128023;159.358738098149;159.728102859405;160.046954227227;160.312221488639;160.521349974904;160.672325664379;160.763694578642;160.794576785101;160.764674871227;160.674276808796;160.524253180566;160.316048796087;160.051668777399;159.733659248606;159.365082815313;158.949489070056;158.490880407788;157.993673480629;157.462656663088;156.908284800231], [156.971389291536;157.430657072004;157.84697804213;158.216342803387;158.535194171208;158.80046143262;159.009589918885;159.16056560836;159.251934522623;159.282816729083;159.252914815208;159.162516752777;159.012493124547;158.804288740068;158.53990872138;158.221899192587;157.853322759294;157.437729014037;156.979120351769;156.48191342461;155.950896607069;155.391183881382;154.808165587067;154.20745650901;153.594841804012;152.976221286573;152.357552610446;151.744793893183;151.143846336199;150.560497392978;150.000365032735;149.468843636298;148.971052045274;148.511784264806;148.095463294681;147.726098533424;147.407247165603;147.144199990631])
      | plot([152.057635404444;152.93604260309;153.834625296826;154.744729643097;155.657590839533;156.564417533794;157.45647648909;158.325176690034;159.162152078811;159.959342124889;160.709069452336;161.404113777147;162.037781442523;162.603969882449;163.097226392739;163.512800643557;163.846690427691;164.095680203997;164.257372064819;164.330208829146;164.313489039122;164.27939575172], [142.228020686971;141.979030910664;141.817339049842;141.744502285515;141.761222075539;141.867337399197;142.061826307913;142.342815767178;142.707599694895;143.152665022428;143.673725527376;144.265763112236;144.923076131425;145.639334301243;146.40763966397;147.220593018964;148.070365181011;148.948772379657;149.847355073393;150.757459419663;151.6703206161;152.055850472277])
      | %plot([116.468514315784;116.438789536125;116.349901463023;116.202706137216;115.998621130155;115.739611892022;115.42817282337;115.067303252679;114.660478551187;114.211616663162;113.725040373958;113.205435679231;112.657806656235;112.087427271827;111.499790591278;110.900555877058;110.29549408704;109.690432297022;109.091197582803;108.503560902254;107.933181517846;107.38555249485;106.865947800123;106.379371510919;105.930509622894;105.523684921402;105.162815350711;104.851376282059;104.592367043926;104.388282036865;104.241086711057;104.152198637956;104.122473858297;104.152198637956;104.241086711057;104.388282036865;104.592367043926;104.851376282059;105.162815350711;105.523684921402;105.930509622894;106.379371510919;106.865947800123;107.38555249485;107.933181517846;108.503560902254;109.091197582803;109.690432297022;110.29549408704;110.900555877058;111.499790591278;112.087427271827;112.657806656235;113.205435679231;113.725040373958;114.211616663162;114.660478551187;115.067303252679;115.42817282337;115.739611892022;115.998621130155;116.202706137216;116.349901463023;116.438789536125;116.468514315784;116.468514315784], [111.618284136057;111.013222346039;110.413987631819;109.826350951271;109.255971566862;108.708342543866;108.188737849139;107.702161559936;107.253299671911;106.846474970419;106.485605399728;106.174166331075;105.915157092943;105.711072085881;105.563876760074;105.474988686973;105.445263907313;105.474988686973;105.563876760074;105.711072085881;105.915157092943;106.174166331075;106.485605399728;106.846474970419;107.253299671911;107.702161559936;108.188737849139;108.708342543866;109.255971566862;109.826350951271;110.413987631819;111.013222346039;111.618284136057;112.223345926075;112.822580640295;113.410217320843;113.980596705252;114.528225728247;115.047830422975;115.534406712178;115.983268600203;116.390093301695;116.750962872386;117.062401941038;117.321411179171;117.525496186232;117.67269151204;117.761579585141;117.7913043648;117.761579585141;117.67269151204;117.525496186232;117.321411179171;117.062401941038;116.750962872386;116.390093301695;115.983268600203;115.534406712178;115.047830422975;114.528225728247;113.980596705252;113.410217320843;112.822580640295;112.223345926075;111.618284136057;111.618284136057])
      | plot([239.23602886498;238.828071429858;237.608127977604;235.587947230552;232.78698463364;229.232214987837;224.957872668068;220.005121927465;214.421660463109;208.261260061133;201.583248745024;194.451939414329;186.936010476274;179.107844435155;171.042830809261;162.818640088593;154.514475725591;146.210311362589;137.986120641921;129.921107016027;122.092940974909;114.577012036853;107.445702706158;100.76769139005;94.607290988073;89.0238295237172;84.0710787831142;79.7967364633452;76.2419668175427;73.4410042206305;71.4208234735788;70.2008800213248;69.7929225862026;70.2008800213248;71.4208234735788;73.4410042206306;76.2419668175428;79.7967364633454;84.0710787831144;89.0238295237174;94.6072909880733;100.76769139005;107.445702706159;114.577012036853;122.092940974909;129.921107016027;137.986120641921;146.210311362589;154.514475725591;162.818640088593;171.042830809261;179.107844435155;186.936010476274;194.451939414329;201.583248745024;208.261260061133;214.421660463109;220.005121927465;224.957872668068;229.232214987837;232.78698463364;235.587947230552;237.608127977604;238.828071429858;239.23602886498;239.23602886498], [155.774275772274;147.47628550917;139.258209428443;131.199192095207;123.376846251889;115.866505365088;108.740498123116;102.067451871182;95.9116316925529;90.3323215006612;85.3832531026163;81.1120887325275;77.5599620381344;74.7610819412943;72.742403187363;71.5233667562631;71.1157126352191;71.5233667562631;72.742403187363;74.7610819412943;77.5599620381345;81.1120887325275;85.3832531026164;90.3323215006612;95.9116316925529;102.067451871182;108.740498123116;115.866505365089;123.376846251889;131.199192095207;139.258209428443;147.47628550917;155.774275772274;164.072266035377;172.290342116104;180.34935944934;188.171705292658;195.682046179459;202.808053421432;209.481099673365;215.636919851994;221.216230043886;226.165298441931;230.43646281202;233.988589506413;236.787469603253;238.806148357184;240.025184788284;240.432838909328;240.025184788284;238.806148357184;236.787469603253;233.988589506413;230.43646281202;226.165298441931;221.216230043886;215.636919851994;209.481099673365;202.808053421432;195.682046179459;188.171705292658;180.34935944934;172.290342116105;164.072266035378;155.774275772274;155.774275772274])
      | plot([252.715889364481;252.243022716633;250.828976737403;248.487369462568;245.240751850236;241.120390602797;236.165967051481;230.425195003451;223.953361231755;216.812793033479;209.072257983804;200.806301666664;192.094529760025;183.020841389688;173.672621134841;164.139897466795;154.514475725591;144.889053984387;135.356330316341;126.008110061494;116.934421691157;108.222649784518;99.9566934673787;92.2161584177032;85.075590219427;78.6037564477313;72.8629843997015;67.9085608483856;63.7881996009461;60.5415819886144;58.199974713779;56.7859287345493;56.3130620867014;56.7859287345493;58.1999747137791;60.5415819886146;63.7881996009463;67.9085608483858;72.8629843997018;78.6037564477315;85.0755902194273;92.2161584177035;99.9566934673791;108.222649784519;116.934421691157;126.008110061494;135.356330316341;144.889053984387;154.514475725591;164.139897466796;173.672621134841;183.020841389688;192.094529760025;200.806301666664;209.072257983803;216.812793033479;223.953361231755;230.425195003451;236.165967051481;241.120390602797;245.240751850236;248.487369462568;250.828976737403;252.243022716633;252.715889364481;252.715889364481], [154.514475725591;144.895228084285;135.36861905618;126.026395093992;116.958526921455;108.252343066071;99.9916888376535;92.2561188521535;85.1201308772245;78.6524483779929;72.9153586725213;67.9641130708855;63.8463947748555;60.6018596625959;58.2617543808809;56.8486154228053;56.3760520890355;56.8486154228053;58.2617543808809;60.6018596625959;63.8463947748555;67.9641130708856;72.9153586725213;78.652448377993;85.1201308772246;92.2561188521536;99.9916888376536;108.252343066072;116.958526921455;126.026395093992;135.36861905618;144.895228084285;154.514475725591;164.133723366898;173.660332395002;183.002556357191;192.070424529728;200.776608385111;209.037262613529;216.772832599029;223.908820573958;230.37650307319;236.113592778661;241.064838380297;245.182556676327;248.427091788587;250.767197070302;252.180336028377;252.652899362147;252.180336028377;250.767197070301;248.427091788587;245.182556676327;241.064838380297;236.113592778661;230.37650307319;223.908820573958;216.772832599029;209.037262613529;200.776608385111;192.070424529728;183.002556357191;173.660332395002;164.133723366898;154.514475725592;154.514475725591])
      | plot([154.514475725591;129.948374815285;179.017586633563;154.514475725591], [240.369848906994;203.583687543869;203.583687543869;240.369848906994])
      | %plot([105.382273904979;149.60125554353], [115.271704271436;156.971085816622])
      | plot([144.688035361469;144.688035361469], [152.057865634561;203.583687543869])
      | plot([164.277926087379;164.277926087379], [152.057865634561;203.583687543869])
      | plot([159.112745895982;159.616665914655], [149.60125554353;149.60125554353])
      | %plot([115.208714269102;159.364705905318], [107.901873998344;149.60125554353])
      | plot([0;311.800511553884;311.800511553884;0;0], [311.800511553884;311.800511553884;0;0;311.800511553884])
      | ;
      | color('red');
      | port_label('LConn', 1,'R')
      | port_label('RConn', 1,'C')
      | port_label('LConn', 2,'Ref')
      | port_label('output', 1,'P')
      | port_label('output', 2,'T')
      | port_label('output', 3,'W')
      | %port_label('RConn', 3,'A')
  Fcn : Fcn  Expr=0.5*((u-1)*(1-n2)+(u+1)*(1-n1))
  Gear Box : fl_lib/Mechanical/Mechanisms/Gear Box  ratio=r  t_in_specify=off  t_in_priority=High  t_in=0 N*m  t_out_specify=off  t_out_priority=High  t_out=0 N*m
  Ideal Rotational Motion Sensor : fl_lib/Mechanical/Mechanical Sensors/Ideal Rotational Motion Sensor  offset=0 rad
  Ideal Torque Source : fl_lib/Mechanical/Mechanical Sources/Ideal Torque Source
  Inertia : fl_lib/Mechanical/Rotational Elements/Inertia  inertia=J kg*m^2  w_specify=on  w_priority=High  w=0 rad/s  t_specify=off  t_priority=High  t=0 N*m
  Product : Product  RndMeth=Zero
  Scope : Scope
      settings: TimeRange=4  YMin=0  YMax=0.014
  Scope1 : Scope
      settings: TimeRange=4  YMin=-0.5005000000000001  YMax=-0.4985000000000001  SaveName=ScopeData2
  Sign : Signum
  Simulink-PS Converter : nesl_utility/Simulink-PS Converter  PhysicalDomain=network_engine_domain  SubClassName=ps_input  LeftPortType=input  RightPortType=output  PseudoPeriodic=off  Frequencies=[]  NoiseDistribution=none  NoiseParameters=[]  Unit=1  AffineConversion=off  InputFiltering=off  SimscapeFilterOrder=1  InputFilterTimeConstant=.001  UdotUserProvided=0
  R : PMIOPort  Port=1  Side=Right
  V : PMIOPort  Tag=PMCPort  Port=2  Side=Left
  Ref : PMIOPort  Tag=PMCPort  Port=3  Side=Left
  wires:
  Capteur de puissance mécanique de rotation/2(C) -> Scope1/1, Product/2
  Fcn/1 -> Product/1
  Product/1 -> Simulink-PS Converter/1, Scope/1
  Sign/1 -> Fcn/1
  Capteur de puissance mécanique de rotation/1(P) -> Sign/1
  connections:
  V/RConn1 -- Capteur de puissance mécanique de rotation/LConn2
  Capteur de puissance mécanique de rotation/LConn1 -- Ideal Torque Source/RConn2 -- Ref/RConn1
  R/RConn1 -- Gear Box/RConn1
  Simulink-PS Converter/RConn1 -- Ideal Torque Source/RConn1
  Gear Box/LConn1 -- Ideal Torque Source/LConn1 -- Capteur de puissance mécanique de rotation/RConn1 -- Inertia/LConn1

== system Library_SII/Mécanique/Roue libre SM ==
  Add1 : Sum
  Constant : Constant  Value=0
  Constant1 : Constant  Value=0
  Constant2 : Constant  Value=inf
  Constante de frottement : Constant  Value=kv
  "Couple constant pour maintenir la roue libre en position \"bloquee\" en l'absence de couple transmis" : Constant  Value=1e-10
  Gain1 : Gain  Gain=-1  SaturateOnIntegerOverflow=on  OutDataTypeStr=Inherit: Same as input  ParamDataTypeStr=Inherit: Same as input
  Joint Stiction Actuator : mblibv1/Sensors &  Actuators/Joint Stiction Actuator  UpdateFromCAD=off  PhysicalDomain=Mechanical  PortType=blob  ActuationStyle=Force  AngleUnits=deg  ArcVelocityUnits=deg/s  ArcAccelerationUnits=deg/s^2  CoordPositionUnits=m  VelocityUnits=m/s  AccelerationUnits=m/s^2  ForceUnits=N  TorqueUnits=N-m  ActiveIO=off  Width=5  DialogClass=EventActuatorBlock  Primitive=R1  FrictionalForceUnits=N  ExternalForceUnits=N  FrictionalTorqueUnits=N*m  ExternalTorqueUnits=N*m  LockingTolerance=1e-2
  Mesures : mblibv1/Sensors &  Actuators/Joint Sensor  UpdateFromCAD=off  PhysicalDomain=Mechanical  PortType=blob  Muxed=off  Pose=off  Angle=off  AngleUnits=deg  ArcVelocity=on  ArcVelocityUnits=rad/s  ArcAcceleration=off  ArcAccelerationUnits=deg/s^2  CoordPosition=on  CoordPositionUnits=m  Velocity=off  VelocityUnits=m/s  Acceleration=off  AccelerationUnits=m/s^2  Quaternion=on  QuaternionDT=off  QuaternionDDT=off  QuaternionUnits=off  OutputVector=[1]  ActiveIO=off  Width=5  DialogClass=MechanicalSensorBlock  Primitive=R1  Force=off  ForceUnits=N  Torque=on  TorqueUnits=N*m  ReferenceFrame=Absolute (World)  ReactionSensedSide=Base  ReactionReferenceFrame=Absolute (World)  ReactionForce=off  ReactionForceUnits=N  ReactionMoment=off  ReactionMomentUnits=N*m
  Product2 : Product  SaturateOnIntegerOverflow=on  InputSameDT=on  OutDataTypeStr=Inherit: Same as first input
  Revolute : mblibv1/Joints/Revolute  LConnTagsString=__newl0|SA1  RConnTagsString=__newr0|SA1  UpdateFromCAD=off  NumSAPorts=2  CutJoint=off  MarkAsCut=off  Primitives=prismatic  PrimitiveProps=R1$World$axe$revolute  DialogClass=JointBlock  R1Axis=axe
  Scope : Scope
      settings: YMin=-0.01  YMax=0.02
  F : PMIOPort  Port=1  Side=Right
  B : PMIOPort  Port=2  Side=Left
  wires:
  Constant1/1 -> Joint Stiction Actuator/3
  "Couple constant pour maintenir la roue libre en position \"bloquee\" en l'absence de couple transmis"/1 -> Add1/2
  Product2/1 -> Joint Stiction Actuator/2
  Mesures/1 -> Gain1/1
  Mesures/2 -> Add1/1, Scope/1  "Couple transmis"
  Gain1/1 -> Product2/2
  Constante de frottement/1 -> Product2/1
  Add1/1 -> Joint Stiction Actuator/4
  Constant2/1 -> Joint Stiction Actuator/5
  Constant/1 -> Joint Stiction Actuator/1
  connections:
  Mesures/LConn1 -- Revolute/LConn2
  Revolute/RConn2 -- Joint Stiction Actuator/RConn1
  F/RConn1 -- Revolute/RConn1
  B/RConn1 -- Revolute/LConn1

== system Library_SII/Signaux/Contrôle de régime ==
  x : Inport
  Clock : Clock
  Constant : Constant  Value=al
  Constant1 : Constant  Value=vl
  Derivative : Derivative
  MATLAB Function : MATLAB Function  TreatAsAtomicUnit=on
  Memory : Memory
  Memory2 : Memory
  Memory5 : Memory
  Transfer Fcn4 : TransferFcn  Denominator=[1/(al*100)^2 2/(al*100) 1]
  xc : Outport
  wires:
  Clock/1 -> Memory5/1, MATLAB Function/1(t)
  Constant/1 -> MATLAB Function/4(al)
  Constant1/1 -> MATLAB Function/5(vl)
  x/1 -> MATLAB Function/3(x)
  Memory5/1 -> MATLAB Function/2(t_1)
  Memory/1 -> MATLAB Function/6(x_1)
  Derivative/1 -> Memory2/1
  MATLAB Function/1(xc) -> Transfer Fcn4/1, Memory/1, Derivative/1
  Memory2/1 -> MATLAB Function/7(v_1)
  Transfer Fcn4/1 -> xc/1

== system Library_SII/Signaux/Frequence-Metre ==
  Signal : Inport
  Constant : Constant  Value=1/Ts
  Constant1 : Constant  Value=spec
  Constant2 : Constant  Value=plage
  Discrete Shift Register : powerlib_extras/Discrete  Control Blocks/Discrete Shift Register  NSamples=N  InitialValue=0  Ts=Ts
  MATLAB Function : MATLAB Function  TreatAsAtomicUnit=on
  Reshape : Reshape  OutputDimensionality=Customize  OutputDimensions=[1,N]
  TsFFT1 : ZeroOrderHold
  Frequence : Outport
  Amplitude : Outport  Port=2
  wires:
  Constant1/1 -> MATLAB Function/3(spec)
  Constant2/1 -> MATLAB Function/4(plage)
  Constant/1 -> MATLAB Function/2(fs)
  MATLAB Function/2(Pmax) -> Amplitude/1
  MATLAB Function/1(F) -> Frequence/1
  Signal/1 -> Discrete Shift Register/1
  TsFFT1/1 -> MATLAB Function/1(x)
  Reshape/1 -> TsFFT1/1
  Discrete Shift Register/1 -> Reshape/1

== system Library_SII/Signaux/Générateur de signal carré ==
  Add1 : Sum
  Step : Step  Time=t  After=a  SampleTime=0
  Step1 : Step  Time=d+t  After=-a  SampleTime=0
  Out1 : Outport
  wires:
  Add1/1 -> Out1/1
  Step1/1 -> Add1/2
  Step/1 -> Add1/1

== system Library_SII/Signaux/Générateur de signal pas ==
  Add1 : Sum
  Ramp : simulink/Sources/Ramp  slope=-p  start=a/p  X0=0
  Ramp1 : simulink/Sources/Ramp  slope=p  start=t  X0=0
  Out1 : Outport
  wires:
  Add1/1 -> Out1/1
  Ramp/1 -> Add1/2
  Ramp1/1 -> Add1/1

== system Library_SII/Signaux/Trapèze ==
  Add : Sum  Inputs=++++
  Ramp : simulink/Sources/Ramp  slope=p  start=t0  X0=0
  Ramp1 : simulink/Sources/Ramp  slope=-p  start=t0+a/p  X0=0
  Ramp2 : simulink/Sources/Ramp  slope=-p  start=t0+th+a/p  X0=0
  Ramp3 : simulink/Sources/Ramp  slope=p  start=t0+th+2*a/p  X0=0
  Out1 : Outport
  wires:
  Ramp3/1 -> Add/4
  Ramp2/1 -> Add/3
  Add/1 -> Out1/1
  Ramp/1 -> Add/1
  Ramp1/1 -> Add/2
